simulink model "gps"  (R2021b)
settings: Solver=VariableStepAuto  StartTime=0.0  StopTime=10.0  RelTol=1e-3
settings Model: Creator=Aazam  LastModifiedBy=Aazam

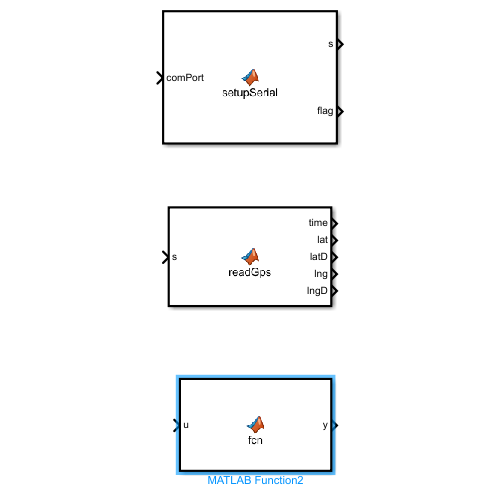
[thumbnail: Simulink's stored preview of the top-level diagram]
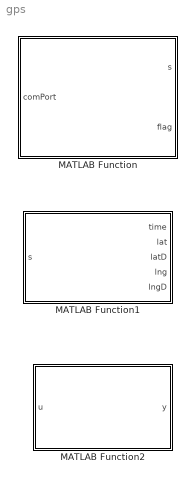
== system gps ==
  MATLAB Function : MATLAB Function  TreatAsAtomicUnit=on
  MATLAB Function1 : MATLAB Function  TreatAsAtomicUnit=on
  MATLAB Function2 : MATLAB Function  TreatAsAtomicUnit=on

== matlab function gps/MATLAB Function1 ==
  data: s input; time output; lat output; latD output; lng output; lngD output
function [time, lat, latD, lng, lngD] = readGps(s)
         % time request
         fprintf(s, 'T');

         %read time
         time = fscanf(s, '%f');

         %latitude req
         fprintf(s, 'A');

         %read lat
         lat = fscanf(s, '%f');

         %sent lat direction request
         fprintf(s, 'a');

         %read Lat direction
         latD = fscanf(s, '%s');

         %send longitude req
         fprintf(s, 'O');

         %read longitude
         lng = fscanf(s, '%f');

         %send longitude direction req
         fprintf(s, 'o');

         %read longitude direction
         lngD = fscanf(s, '%s');
end

== matlab function gps/MATLAB Function ==
  data: comPort input; s output; flag output
% https://www.youtube.com/watch?v=Ct8NCOTk2lM

function [s, flag] = setupSerial(comPort)

s = serial(comPort);
set(s, 'DataBits', 8);
set(s, 'StopBits', 1);
set(s, 'BaudRate', 9600);
set(s, 'Parity', 'none');
fopen(s);

c = 'b';
while (c ~= 'c')
    c = fread(s, 1, 'uchar');
end

if (c == 'c')
    disp('serial read');
end

fprintf(s, '%c', 'c');
flag = 1;
disp('Serial Communication setup.');
fscanf(s, '%u');

end

== matlab function gps/MATLAB Function2 ==
  data: u input; y output
function y = fcn(u)
comPort = '/dev/';

if (~exist('serialFlag', 'var'))
    [arduino.s, serialFlag] = setupSerial(comPort);
end


while (true)

    [time, lat, latD, lng, lngD] = readGps(arduino.s);

    fprintf('Time: %f\n', time);
    fprintf('Lat: %f%s\n', lat, latD);
    fprintf('Long: %f%s\n', lng, lngD);

    pause(0.5);

end
